simulink model "L2_3_mux_scope"  (R2025b)
settings: Solver=VariableStepAuto  StartTime=0.0  StopTime=5  RelTol=1e-3
libraries: simulink x1
settings Model: Creator=kimsteph  LastModifiedBy=kimsteph

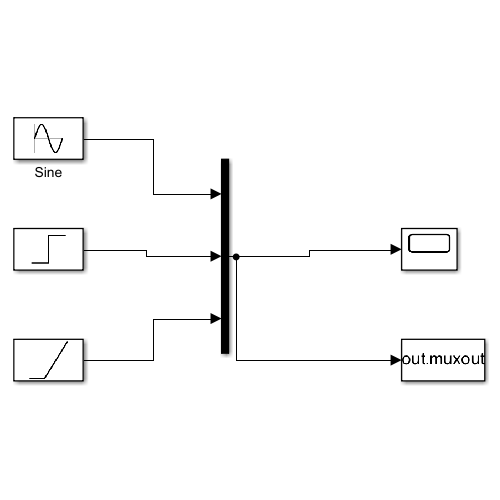
[thumbnail: Simulink's stored preview of the top-level diagram]
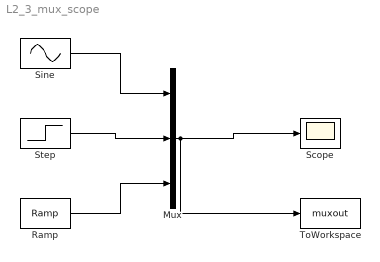
== system L2_3_mux_scope ==
  Mux : Mux  Inputs=3
  Ramp : simulink/Sources/Ramp  slope=0.5  start=0  InitialOutput=0
  Scope : Scope
  Sine : Sin  Frequency=2*pi  SampleTime=0
  Step : Step  Time=2  SampleTime=0
  ToWorkspace : ToWorkspace  VariableName=muxout  SaveFormat=Timeseries  SampleTime=-1
  wires:
  Sine/1 -> Mux/1
  Step/1 -> Mux/2
  Ramp/1 -> Mux/3
  Mux/1 -> Scope/1, ToWorkspace/1
